simulink model "MultiSiteSimpleFeatureDetector"  (R2016b)
settings: Solver=FixedStepDiscrete  StartTime=0.0  StopTime=inf  FixedStep=sCoreParams.core.stepPeriod  RelTol=1e-3
undefined symbols (not defined in the file): sCoreParams, sCoreParams_decoders_txDetector_anyAll, sCoreParams_decoders_txDetector_detectChannelInds, sCoreParams_decoders_txDetector_nDetectionsRequested, sCoreParams_decoders_txDetector_ProbabilityOfStim, sCoreParams_decoders_txDetector_txRMS, sCoreParams_decoders_txDetector_txRMSLower, sCoreParams_decoders_txDetector_txSign, sCoreParams_stimulator_possibleStimRealChannelNumbers
libraries: simulink x1, dspswit3 x1, dspsigops x1
settings Model: DataTypeOverride=Double  MinMaxOverflowLogging=ForceOff  Creator=anish  LastModifiedBy=rzelmann
settings SolverCC: EnableConcurrentExecution=on
settings DataIOCC: SaveFormat=StructureWithTime  SignalLoggingSaveFormat=ModelDataLogs  SaveOutput=off  SignalLogging=off  DSMLogging=off  SaveTime=off
settings OptimizationCC: BlockReduction=off  ConditionallyExecuteInputs=off  DefaultParameterBehavior=Inlined  OptimizeBlockIOStorage=off  BufferReuse=off  GlobalBufferReuse=off  ExpressionFolding=off  LocalBlockOutputs=off  LifeSpan=inf
settings DebuggingCC: SignalRangeChecking=error  SaveWithParameterizedLinksMsg=none  MultiTaskDSMMsg=warning  MultiTaskCondExecSysMsg=none  AllowSymbolicDim=off  ModelReferenceSymbolNameMessage=none  StateNameClashWarn=warning  SFUnexpectedBacktrackingDiag=warning  SFNoUnconditionalDefaultTransitionDiag=warning  SFExecutionAtInitializationDiag=none
settings HardwareCC: ProdBitPerPointer=32  ProdBitPerSizeT=32  ProdBitPerPtrDiffT=32  ProdLargestAtomicFloat=None  ProdWordSize=32  ProdLongLongMode=on  ProdHWDeviceType=Generic->32-bit x86 compatible  TargetBitPerPointer=64  TargetLargestAtomicFloat=Float  TargetLongLongMode=on  TargetIntDivRoundTo=Zero  TargetEndianess=LittleEndian  TargetWordSize=64  TargetHWDeviceType=Intel->x86-64 (Windows64)
settings ModelReferenceCC: UpdateModelReferenceTargets=Force  ModelReferenceNumInstancesAllowed=Single  ModelReferencePassRootInputsByReference=off
settings RTWCC: SystemTargetFile=slrt.tlc  TemplateMakefile=slrt_default_tmf  Description=Simulink Real-Time  BuildConfiguration=Faster Runs  RTWCompilerOptimization=on
settings ConfigComp: CovMetricSettings=dw  CovHtmlReporting=on  CovSaveCumulativeToWorkspaceVar=on  CovSaveSingleToWorkspaceVar=on  CovExternalEMLEnable=off  CovSFcnEnable=off

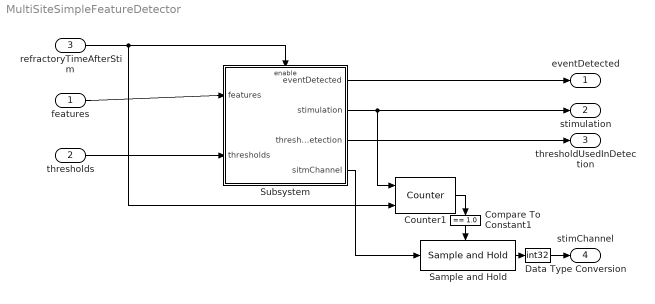
== system MultiSiteSimpleFeatureDetector ==
  features : Inport  PortDimensions=[1 sCoreParams.decoders.txDetector.nFeatures]  SampleTime=sCoreParams.core.stepPeriod
  thresholds : Inport  Port=2  PortDimensions=[1 sCoreParams.decoders.txDetector.nFeatures]  SampleTime=sCoreParams.core.stepPeriod
  refractoryTimeAfterStim : Inport  Port=3  OutDataTypeStr=boolean  SampleTime=sCoreParams.core.stepPeriod
  Compare To Constant1 : simulink/Logic and Bit Operations/Compare To Constant  relop===  const=1.0  OutDataTypeStr=boolean
  Counter1 : dspswit3/Counter  Direction=Up  CountEvent=Rising edge  CounterSize=User defined  MaxCount=1024  InitialCount=0  Output=Count  HitValue=1  ResetInput=on  SamplesPerFrame=1  Ts=1  CntDtype=double  HitDtype=Logical
  Data Type Conversion : DataTypeConversion  OutDataTypeStr=int32
  Sample and Hold : dspsigops/Sample and Hold  trig=Rising edge  initCond=0  latchinput=off
  Subsystem : Subsystem
  eventDetected : Outport  SampleTime=sCoreParams.core.stepPeriod
  stimulation : Outport  Port=2  SampleTime=sCoreParams.core.stepPeriod
  thresholdUsedInDetection : Outport  Port=3  SampleTime=sCoreParams.core.stepPeriod
  stimChannel : Outport  Port=4  OutDataTypeStr=int32
  wires:
  features/1 -> Subsystem/1(features)
  thresholds/1 -> Subsystem/2(thresholds)
  Subsystem/1(eventDetected) -> eventDetected/1
  Subsystem/3(thresholdUsedInDetection) -> thresholdUsedInDetection/1
  Subsystem/2(stimulation) -> Counter1/1, stimulation/1
  refractoryTimeAfterStim/1 -> Counter1/2, Subsystem/Enable
  Subsystem/4(sitmChannel) -> Sample and Hold/1
  Data Type Conversion/1 -> stimChannel/1
  Sample and Hold/1 -> Data Type Conversion/1
  Counter1/1 -> Compare To Constant1/1
  Compare To Constant1/1 -> Sample and Hold/Trigger

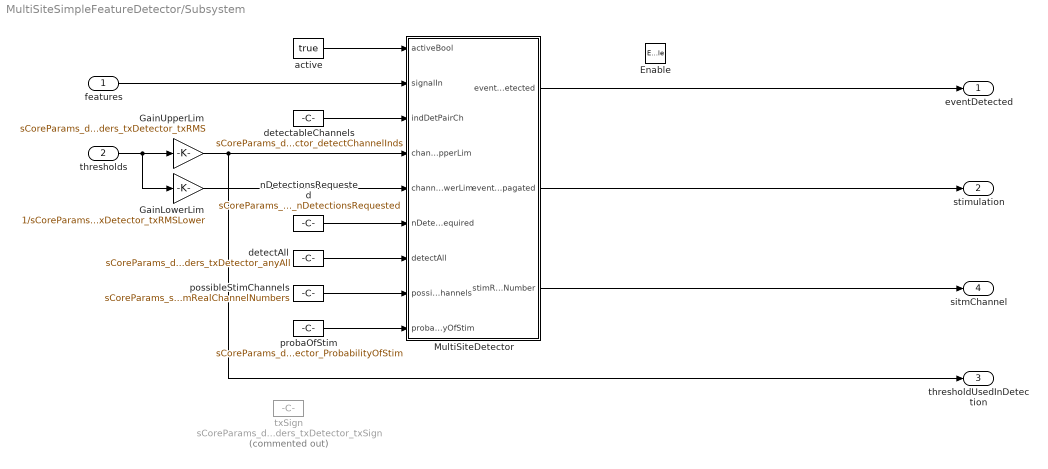
== system MultiSiteSimpleFeatureDetector/Subsystem ==
  features : Inport
  thresholds : Inport  Port=2
  Enable : EnablePort
  GainLowerLim : Gain  Gain=1/sCoreParams_decoders_txDetector_txRMSLower
  GainUpperLim : Gain  Gain=sCoreParams_decoders_txDetector_txRMS
  MultiSiteDetector : MATLAB Function  TreatAsAtomicUnit=on
  active : Constant  Value=true
  detectAll : Constant  Value=sCoreParams_decoders_txDetector_anyAll
  detectableChannels : Constant  Value=sCoreParams_decoders_txDetector_detectChannelInds
  nDetectionsRequested : Constant  Value=sCoreParams_decoders_txDetector_nDetectionsRequested
  possibleStimChannels : Constant  Value=sCoreParams_stimulator_possibleStimRealChannelNumbers
  probaOfStim : Constant  Value=sCoreParams_decoders_txDetector_ProbabilityOfStim
  txSign : Constant  Commented=on  Value=sCoreParams_decoders_txDetector_txSign
  eventDetected : Outport
  stimulation : Outport  Port=2
  thresholdUsedInDetection : Outport  Port=3
  sitmChannel : Outport  Port=4
  wires:
  MultiSiteDetector/2(eventPropagated) -> stimulation/1
  GainUpperLim/1 -> MultiSiteDetector/4(channelThresholdUpperLim), thresholdUsedInDetection/1
  thresholds/1 -> GainLowerLim/1, GainUpperLim/1
  active/1 -> MultiSiteDetector/1(activeBool)
  nDetectionsRequested/1 -> MultiSiteDetector/6(nDetectionsRequired)
  MultiSiteDetector/1(eventDetected) -> eventDetected/1
  detectableChannels/1 -> MultiSiteDetector/3(indDetPairCh)
  features/1 -> MultiSiteDetector/2(signalIn)
  detectAll/1 -> MultiSiteDetector/7(detectAll)
  probaOfStim/1 -> MultiSiteDetector/9(probabilityOfStim)
  MultiSiteDetector/3(stimRealChannelNumber) -> sitmChannel/1
  possibleStimChannels/1 -> MultiSiteDetector/8(possibleStimChannels)
  GainLowerLim/1 -> MultiSiteDetector/5(channelThresholdLowerLim)

== matlab function MultiSiteSimpleFeatureDetector/Subsystem/MultiSiteDetector ==
  data: activeBool input; eventDetected output; signalIn input; indDetPairCh input; channelThresholdUpperLim input; channelThresholdLowerLim input; nDetectionsRequired input; eventPropagated output; detectAll input; stimRealChannelNumber output; possibleStimChannels input; probabilityOfStim input
function [eventDetected, eventPropagated, stimRealChannelNumber] = MultiSiteDetector(activeBool, signalIn, indDetPairCh, channelThresholdUpperLim, channelThresholdLowerLim, nDetectionsRequired, detectAll, possibleStimChannels, probabilityOfStim)
%#codegen
% uses MultiSiteCoherenceDetectorAll_EML.m - it should actually be called MultiSiteDetectorAll_EML
if (detectAll >= 1) % 1 means ALL - 0 means ANY
    [eventDetected, eventPropagated, stimRealChannelNumber] = MultiSiteCoherenceDetectorAll_EML(activeBool, signalIn, indDetPairCh, channelThresholdUpperLim, channelThresholdLowerLim, nDetectionsRequired, possibleStimChannels, probabilityOfStim);
else
    [eventDetected, eventPropagated, stimRealChannelNumber] = MultiSiteCoherenceDetectorAny_EML(activeBool, signalIn, indDetPairCh, channelThresholdUpperLim, channelThresholdLowerLim, nDetectionsRequired, possibleStimChannels, probabilityOfStim);
end
